simulink model "lab_7_simulink_part2"  (R2021b)
settings: Solver=VariableStepAuto  StartTime=0.0  StopTime=20  RelTol=1e-3
settings Model: Creator=rcmas  LastModifiedBy=rcmas

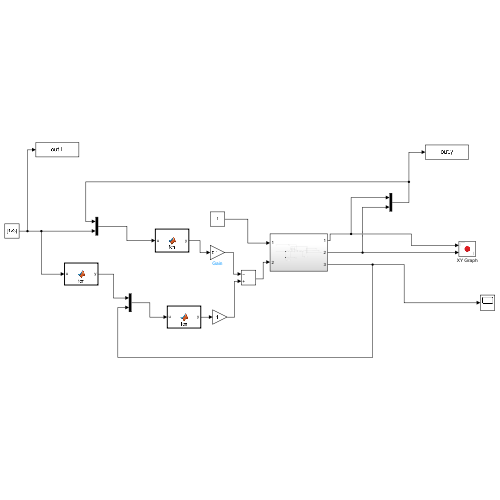
[thumbnail: Simulink's stored preview of the top-level diagram]
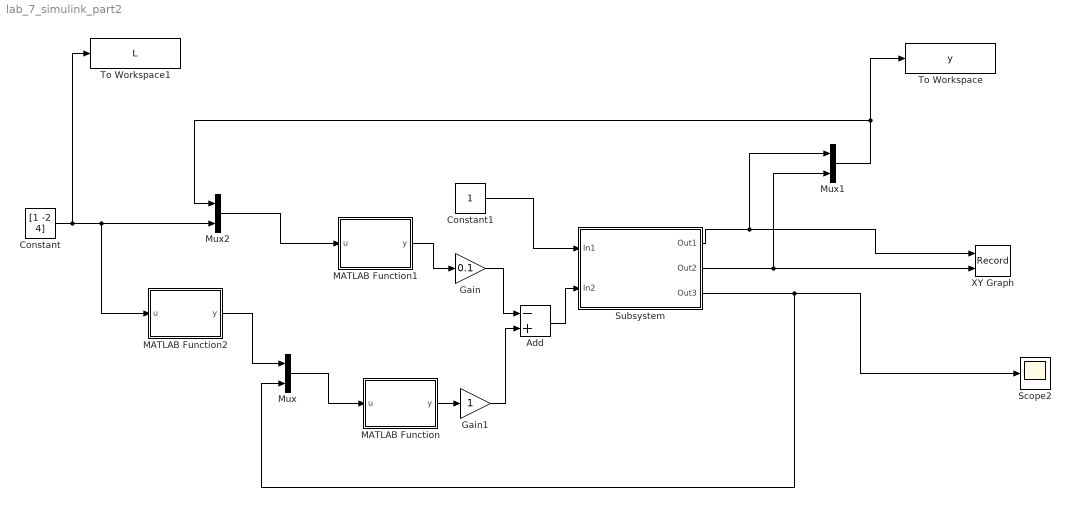
== system lab_7_simulink_part2 ==
  Add : Sum  Inputs=-+
  Constant : Constant  Value=[1 -2 4]
  Constant1 : Constant
  Gain : Gain  Gain=0.1
  Gain1 : Gain
  MATLAB Function : MATLAB Function  TreatAsAtomicUnit=on
  MATLAB Function1 : MATLAB Function  Tag=sqrt  TreatAsAtomicUnit=on
  MATLAB Function2 : MATLAB Function  TreatAsAtomicUnit=on
  Mux : Mux  Inputs=2
  Mux1 : Mux  Inputs=2
  Mux2 : Mux  Inputs=2
  Scope2 : Scope
  Subsystem : Subsystem
  To Workspace : ToWorkspace  VariableName=y  SaveFormat=Timeseries  SampleTime=-1
  To Workspace1 : ToWorkspace  VariableName=L  SaveFormat=Timeseries  SampleTime=-1
  XY Graph : Record  FileSettingsInternal="{\"entries\":[{\"content\":{\"excelSettings\":{\"content\":{},\"type\":\"Streamout.ExcelSettings\"}},\"type\":\"Streamout.FileSettingStorage\",\"uuid\":\"9c0d3076-a6f9-459c-8c44-b24a2157b0ee\"}],\"packageUris\":[\"http://schema.mathworks.com/mf0/streamout_blocks/R2020a\"],\"version\":\"1.0\"}"  Layout=[1 1]  SignalsInternal="{\"entries\":[{\"content\":{\"signals\":[{\"content\":{\"blockPath\":[\"lab_7_simulink_part2/XY Graph\"],\"channel\":[],\"dimensions\":[1],\"domain\":\"lab_7_simulink_part2/XY Graph\",\"lineColor\":\"#a2142f\",\"plots\":[1],\"port\":1,\"sid\":[\"\"],\"signalID\":408,\"signalName\":\"Subsystem:1\"},\"type\":\"RecordBlkView.Signal\",\"uuid\":\"72b0f34d-1a2e-4248-b2e2-52b6cfd00c93\"},{\"content\":{\"blockPath\":[\"lab_7_simulink_part2/XY Graph\"],\"channel\":[],\"dimensions\":[1],\"domain\":\"lab_7_simulink_part2/XY Graph\",\"lineColor\":\"#139fff\",\"plots\":[1],\"port\":2,\"sid\":[\"\"],\"signalID\":412,\"signalName\":\"Subsystem:2\"},\"type\":\"RecordBlkView.Signal\",\"uuid\":\"a3b1e577-0433-4d18-ab8c-2d1e4971d592\"}]},\"type\":\"RecordBlkView.InputSignals\",\"uuid\":\"68814cb5-4627-424d-9e28-7970ac121390\"}],\"packageUris\":[\"http://schema.mathworks.com/mf0/streamout_blocks/R2020a\"],\"version\":\"1.0\"}"  VisualizationBindings="{\"xyplotplugin\":{\"info\":[{\"series\":[{\"bindingParametersList\":[{\"parameter\":\"X-Axis\",\"signalID\":408,\"signalName\":\"Subsystem:1\"},{\"parameter\":\"Y-Axis\",\"signalID\":412,\"signalName\":\"Subsystem:2\"}],\"seriesID\":11607}],\"subplotID\":1}]}}"  CompatibilityTag=XY
  wires:
  Subsystem/1(Out1) -> Mux1/1, XY Graph/1
  Subsystem/2(Out2) -> Mux1/2, XY Graph/2
  Subsystem/3(Out3) -> Mux/2, Scope2/1
  Mux/1 -> MATLAB Function/1(u)
  MATLAB Function2/1(y) -> Mux/1
  MATLAB Function1/1(y) -> Gain/1
  MATLAB Function/1(y) -> Gain1/1
  Constant/1 -> MATLAB Function2/1(u), Mux2/2, To Workspace1/1
  Mux1/1 -> To Workspace/1, Mux2/1
  Gain1/1 -> Add/2
  Add/1 -> Subsystem/2(In2)
  Gain/1 -> Add/1
  Constant1/1 -> Subsystem/1(In1)
  Mux2/1 -> MATLAB Function1/1(u)

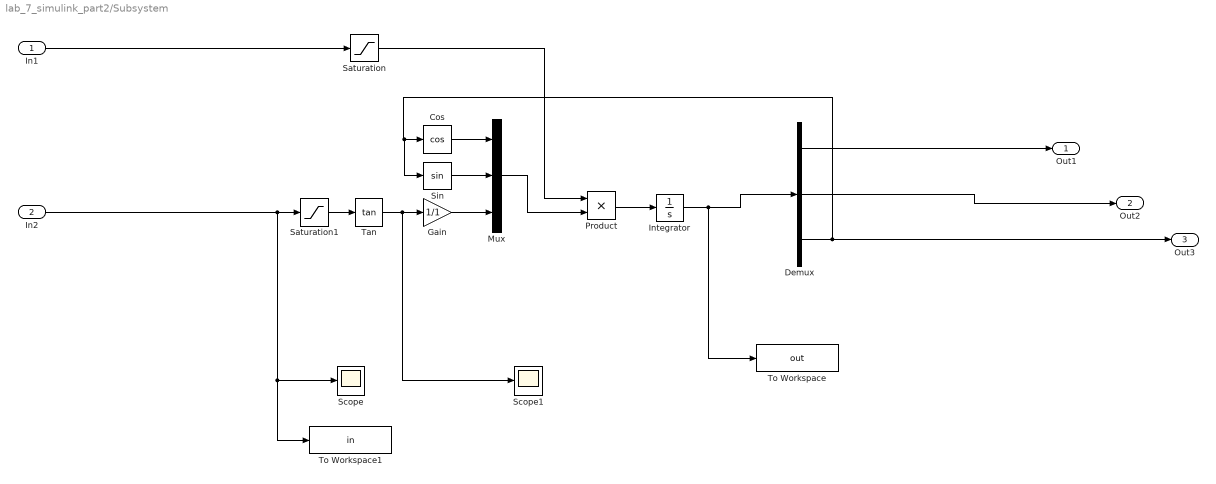
== system lab_7_simulink_part2/Subsystem ==
  In1 : Inport
  In2 : Inport  Port=2
  Cos : Trigonometry  Operator=cos
  Demux : Demux  Outputs=3
  Gain : Gain  Gain=1/1
  Integrator : Integrator  InitialCondition=[8 5 pi/2]
  Mux : Mux  Inputs=3
  Product : Product
  Saturation : Saturate  UpperLimit=1  LowerLimit=-1
  Saturation1 : Saturate  UpperLimit=1  LowerLimit=-1
  Scope : Scope
  Scope1 : Scope
  Sin : Trigonometry
  Tan : Trigonometry  Operator=tan
  To Workspace : ToWorkspace  VariableName=out  SaveFormat=Timeseries  SampleTime=-1
  To Workspace1 : ToWorkspace  VariableName=in  SaveFormat=Timeseries  SampleTime=-1
  Out1 : Outport
  Out2 : Outport  Port=2
  Out3 : Outport  Port=3
  wires:
  Demux/1 -> Out1/1
  In1/1 -> Saturation/1
  Gain/1 -> Mux/3
  In2/1 -> To Workspace1/1, Scope/1, Saturation1/1
  Tan/1 -> Scope1/1, Gain/1
  Sin/1 -> Mux/2
  Saturation/1 -> Product/1
  Saturation1/1 -> Tan/1
  Mux/1 -> Product/2
  Integrator/1 -> To Workspace/1, Demux/1
  Demux/2 -> Out2/1
  Demux/3 -> Out3/1, Sin/1, Cos/1
  Product/1 -> Integrator/1
  Cos/1 -> Mux/1

== matlab function lab_7_simulink_part2/MATLAB Function ==
  data: u input; y output
function y = fcn(u)

y = angdiff(u(2), u(1));

== matlab function lab_7_simulink_part2/MATLAB Function2 ==
  data: u input; y output
function y = fcn(u)

y = atan2(-u(1), u(2));

== matlab function lab_7_simulink_part2/MATLAB Function1 ==
  data: u input; y output
function y = fcn(u)
x = u(1);
y = u(2);
a = u(3);
b = u(4);
c = u(5);
y = (a*x + b*y +c)/sqrt(a^2 +b^2);
